simulink model "dsp_proj_v3"  (R2025b)
settings: Solver=FixedStepDiscrete  StartTime=0.0  StopTime=1e-4  FixedStep=1/60e6  RelTol=1e-3
libraries: hdlsllib x12, simulink x4, dspfdesign x3
settings Model: Creator=UTSAB KARAN  LastModifiedBy=souma

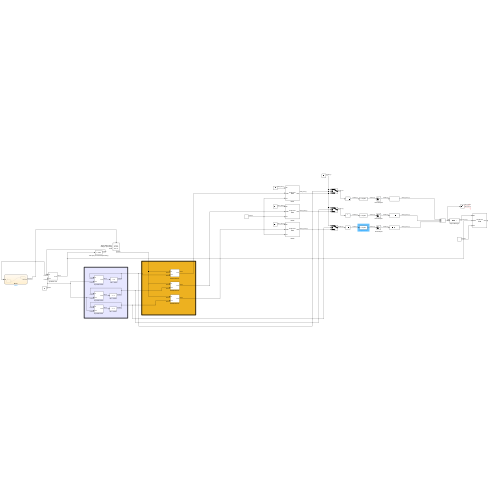
[thumbnail: Simulink's stored preview of the top-level diagram]
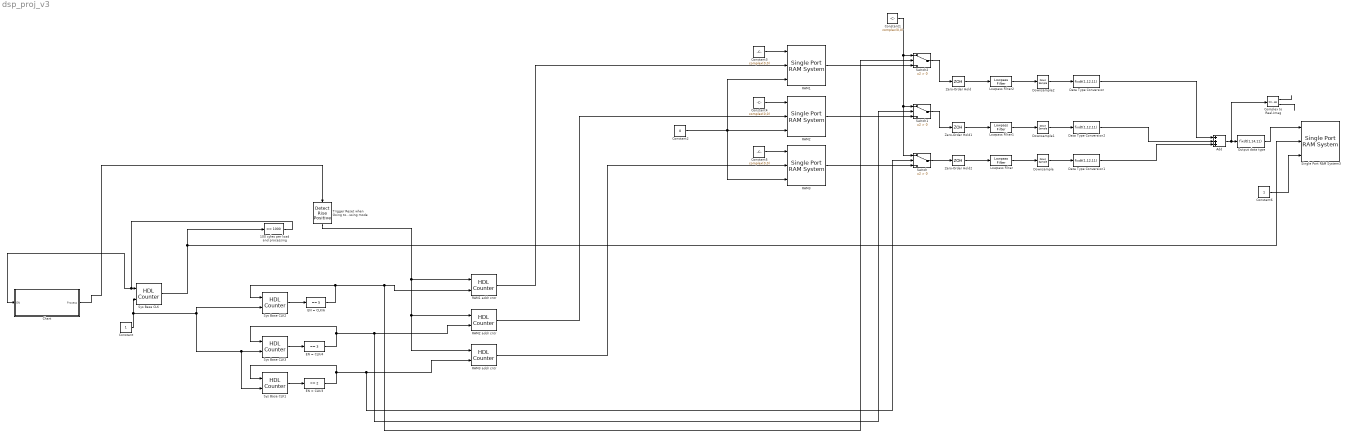
== system dsp_proj_v3 ==
  100 cyles per load and processing : simulink/Logic and Bit Operations/Compare To Constant  relop===  const=1000  OutDataTypeStr=boolean
  Add : Sum  Inputs=+++
  Chart : Stateflow chart  TreatAsAtomicUnit=on
  Complex to Real-Imag : ComplexToRealImag
  Constant : Constant  OutDataTypeStr=boolean
  Constant1 : Constant  Value=complex(0,0)  VectorParams1D=off  SampleTime=-1  LockScale=on
  Constant2 : Constant  Value=0  OutDataTypeStr=boolean
  Constant3 : Constant  Value=complex(0,0)  OutDataTypeStr=fixdt(1,8,6)
  Constant4 : Constant  Value=complex(0,0)  OutDataTypeStr=fixdt(1,10,8)
  Constant5 : Constant  Value=complex(0,0)  OutDataTypeStr=fixdt(1,12,10)
  Constant6 : Constant  OutDataTypeStr=boolean
  Data Type Conversion : DataTypeConversion  OutDataTypeStr=fixdt(1,12,11)  RndMeth=Floor
  Data Type Conversion1 : DataTypeConversion  OutDataTypeStr=fixdt(1,12,11)  RndMeth=Floor
  Data Type Conversion2 : DataTypeConversion  OutDataTypeStr=fixdt(1,12,11)  RndMeth=Floor
  Downsample : DownSample  RateOptions=Allow multirate processing
  Downsample1 : DownSample  RateOptions=Allow multirate processing
  Downsample2 : DownSample  RateOptions=Allow multirate processing
  EN = CLK/3 : simulink/Logic and Bit Operations/Compare To Constant  relop===  const=2  OutDataTypeStr=boolean
  EN = CLK/4 : simulink/Logic and Bit Operations/Compare To Constant  relop===  const=3  OutDataTypeStr=boolean
  EN = CLK/6 : simulink/Logic and Bit Operations/Compare To Constant  relop===  const=5  OutDataTypeStr=boolean
  Lowpass Filter : dspfdesign/Lowpass Filter  FilterType=FIR  DesignForMinimumOrder=on  FilterOrder=50  PassbandFrequency=12e6  StopbandFrequency=25e6  PassbandRipple=0.1  StopbandAttenuation=80  SampleRateMode=Specify on dialog  SampleRate=60e6  SimulateUsing=Interpreted execution  roundingMode=Floor  coeffsDataTypeStr=fixdt(1,16,15)
  Lowpass Filter1 : dspfdesign/Lowpass Filter  FilterType=FIR  DesignForMinimumOrder=on  FilterOrder=50  PassbandFrequency=10e6  StopbandFrequency=20e6  PassbandRipple=0.1  StopbandAttenuation=80  SampleRateMode=Specify on dialog  SampleRate=60e6  SimulateUsing=Interpreted execution  roundingMode=Floor  coeffsDataTypeStr=fixdt(1,16,15)
  Lowpass Filter2 : dspfdesign/Lowpass Filter  FilterType=FIR  DesignForMinimumOrder=on  FilterOrder=50  PassbandFrequency=7.5e6  StopbandFrequency=15e6  PassbandRipple=0.1  StopbandAttenuation=80  SampleRateMode=Specify on dialog  SampleRate=60e6  SimulateUsing=Interpreted execution  roundingMode=Floor  coeffsDataTypeStr=fixdt(1,16,15)
  Output data type : DataTypeConversion  OutDataTypeStr=fixdt(1,14,11)  SaturateOnIntegerOverflow=off  RndMeth=Floor  LockScale=on
  RAM1 : hdlsllib/HDL RAMs/Single Port RAM System  RAMType=Single port  AsyncRead=off  WriteOutputValue=New data  RAMInitialValue=ram1_init_data  allowBusInputs=off  WritesHaveOutput=on  NumReads=0  NumWrites=1  SimulateUsing=Code generation  ModelRAMDelay=on  VectorAccess=Parallel
  RAM1 addr cntr : hdlsllib/Sources/HDL Counter  CountType=Count limited  CountInit=0  CountStep=1  CountMax=3000  CountFromType=Initial value  CountFrom=0  CountResetPort=on  CountLoadPort=off  CountEnbPort=on  CountDirPort=off  CountHitOutputPort=off  CountDataType=Unsigned  CountWordLen=12  CountFracLen=0  CountSampTime=1
  RAM2 : hdlsllib/HDL RAMs/Single Port RAM System  RAMType=Single port  AsyncRead=off  WriteOutputValue=New data  RAMInitialValue=ram2_init_data  allowBusInputs=off  WritesHaveOutput=on  NumReads=0  NumWrites=1  SimulateUsing=Code generation  ModelRAMDelay=on  VectorAccess=Parallel
  RAM2 addr cntr : hdlsllib/Sources/HDL Counter  CountType=Count limited  CountInit=0  CountStep=1  CountMax=3000  CountFromType=Initial value  CountFrom=0  CountResetPort=on  CountLoadPort=off  CountEnbPort=on  CountDirPort=off  CountHitOutputPort=off  CountDataType=Unsigned  CountWordLen=12  CountFracLen=0  CountSampTime=1
  RAM3 : hdlsllib/HDL RAMs/Single Port RAM System  RAMType=Single port  AsyncRead=off  WriteOutputValue=New data  RAMInitialValue=ram3_init_data  allowBusInputs=off  WritesHaveOutput=on  NumReads=0  NumWrites=1  SimulateUsing=Code generation  ModelRAMDelay=on  VectorAccess=Parallel
  RAM3 addr cntr : hdlsllib/Sources/HDL Counter  CountType=Count limited  CountInit=0  CountStep=1  CountMax=3000  CountFromType=Initial value  CountFrom=0  CountResetPort=on  CountLoadPort=off  CountEnbPort=on  CountDirPort=off  CountHitOutputPort=off  CountDataType=Unsigned  CountWordLen=12  CountFracLen=0  CountSampTime=1
  Single Port RAM System3 : hdlsllib/HDL RAMs/Single Port RAM System  RAMType=Single port  AsyncRead=off  WriteOutputValue=New data  RAMInitialValue=0  allowBusInputs=off  WritesHaveOutput=on  NumReads=0  NumWrites=1  SimulateUsing=Code generation  ModelRAMDelay=on  VectorAccess=Parallel
  Switch : Switch  Criteria=u2 > Threshold  SaturateOnIntegerOverflow=off  InputSameDT=off
  Switch1 : Switch  Criteria=u2 > Threshold  SaturateOnIntegerOverflow=off  InputSameDT=off
  Switch2 : Switch  Criteria=u2 > Threshold  SaturateOnIntegerOverflow=off  InputSameDT=off
  Sys Base CLK : hdlsllib/Sources/HDL Counter  CountType=Count limited  CountInit=0  CountStep=1  CountMax=1000  CountFromType=Initial value  CountFrom=0  CountResetPort=on  CountLoadPort=off  CountEnbPort=on  CountDirPort=off  CountHitOutputPort=off  CountDataType=Unsigned  CountWordLen=12  CountFracLen=0  CountSampTime=1
  Sys Base CLK1 : hdlsllib/Sources/HDL Counter  CountType=Count limited  CountInit=0  CountStep=1  CountMax=2  CountFromType=Initial value  CountFrom=0  CountResetPort=on  CountLoadPort=off  CountEnbPort=on  CountDirPort=off  CountHitOutputPort=off  CountDataType=Unsigned  CountWordLen=12  CountFracLen=0  CountSampTime=1
  Sys Base CLK2 : hdlsllib/Sources/HDL Counter  CountType=Count limited  CountInit=0  CountStep=1  CountMax=5  CountFromType=Initial value  CountFrom=0  CountResetPort=on  CountLoadPort=off  CountEnbPort=on  CountDirPort=off  CountHitOutputPort=off  CountDataType=Unsigned  CountWordLen=12  CountFracLen=0  CountSampTime=1
  Sys Base CLK3 : hdlsllib/Sources/HDL Counter  CountType=Count limited  CountInit=0  CountStep=1  CountMax=3  CountFromType=Initial value  CountFrom=0  CountResetPort=on  CountLoadPort=off  CountEnbPort=on  CountDirPort=off  CountHitOutputPort=off  CountDataType=Unsigned  CountWordLen=12  CountFracLen=0  CountSampTime=1
  Trigger Reset when Going to processing mode : hdlsllib/Logic and Bit Operations/Detect Rise Positive  vinit=0  OutDataTypeStr=boolean
  Zero-Order Hold : ZeroOrderHold  SampleTime=1/10e6
  Zero-Order Hold1 : ZeroOrderHold  SampleTime=1/15e6
  Zero-Order Hold2 : ZeroOrderHold  SampleTime=1/20e6
  wires:
  Sys Base CLK/1 -> Single Port RAM System3/2, 100 cyles per load and processing/1
  Constant/1 -> Sys Base CLK3/2, Sys Base CLK1/2, Sys Base CLK2/2, Sys Base CLK/2
  100 cyles per load and processing/1 -> Chart/1(EN), Sys Base CLK/1
  EN = CLK/3/1 -> Sys Base CLK1/1, RAM3 addr cntr/2, Switch/2
  Switch1/1 -> Zero-Order Hold1/1
  Add/1 -> Complex to Real-Imag/1, Output data type/1
  Output data type/1 -> Single Port RAM System3/1
  Chart/1(Process) -> Trigger Reset when Going to processing mode/1
  Trigger Reset when Going to processing mode/1 -> RAM1 addr cntr/1, RAM3 addr cntr/1, RAM2 addr cntr/1
  RAM1/1 -> Switch2/3
  Constant1/1 -> Switch/1, Switch1/1, Switch2/1
  RAM1 addr cntr/1 -> RAM1/2
  RAM2 addr cntr/1 -> RAM2/2
  Sys Base CLK1/1 -> EN = CLK/3/1
  Sys Base CLK2/1 -> EN = CLK/6/1
  EN = CLK/4/1 -> Sys Base CLK3/1, RAM2 addr cntr/2, Switch1/2
  Sys Base CLK3/1 -> EN = CLK/4/1
  RAM3 addr cntr/1 -> RAM3/2
  Constant2/1 -> RAM1/3, RAM2/3, RAM3/3
  EN = CLK/6/1 -> RAM1 addr cntr/2, Switch2/2, Sys Base CLK2/1
  RAM2/1 -> Switch1/3
  RAM3/1 -> Switch/3
  Switch/1 -> Zero-Order Hold2/1
  Switch2/1 -> Zero-Order Hold/1
  Lowpass Filter2/1 -> Downsample2/1
  Lowpass Filter1/1 -> Downsample1/1
  Lowpass Filter/1 -> Downsample/1
  Zero-Order Hold/1 -> Lowpass Filter2/1
  Zero-Order Hold1/1 -> Lowpass Filter1/1
  Zero-Order Hold2/1 -> Lowpass Filter/1
  Downsample2/1 -> Data Type Conversion/1
  Downsample1/1 -> Data Type Conversion2/1
  Downsample/1 -> Data Type Conversion1/1
  Data Type Conversion1/1 -> Add/3
  Data Type Conversion2/1 -> Add/2
  Data Type Conversion/1 -> Add/1
  Constant5/1 -> RAM3/1
  Constant4/1 -> RAM2/1
  Constant3/1 -> RAM1/1
  Constant6/1 -> Single Port RAM System3/3
  Complex to Real-Imag/1 -> ?
  Complex to Real-Imag/2 -> ?

== stateflow chart dsp_proj_v3/Chart ==
  settings: stateMachineType=MOORE_MACHINE  executeAtInitialization=1
  state Processing
    Process = true
  state Data_Loading
    Process = false
  Data_Loading -> Processing : [ EN==1]
  (default) -> Data_Loading
  data: Process output; EN input
